simulink model "power_supply"  (R2023b)
settings: Solver=ode1  StartTime=0.0  StopTime=0.16  FixedStep=Ts  MaxStep=1e-6  RelTol=1e-4  EnableMultiTasking=on
values from neighbouring files (symbols this model uses):
  ca = 36e-6    (= 3.6e-05)    [parameters.m]
  cd = 2000e-6    (= 0.002)    [parameters.m]
  ckz = 1.2e-6    (= 1.2e-06)    [parameters.m]
  cs = 7720e-6    (= 0.00772)    [parameters.m]
  E = 512    [parameters.m]
  Kp1 = 0.2    [parameters.m]
  Kp2 = 2.22    [parameters.m]
  La = 0.1e-3    (= 0.0001)    [parameters.m]
  Ld = 0.3e-3    (= 0.0003)    [parameters.m]
  Lk = 2e-3    (= 0.002)    [parameters.m]
  Lm2 = 21e-3    (= 0.021)    [parameters.m]
  Ls = 0.7e-3    (= 0.0007)    [parameters.m]
  Ra = 0.01    [parameters.m]
  Rk = 19.2    [parameters.m]
  Rm2 = 20    [parameters.m]
  Rs = 0.12    [parameters.m]
  Vref = 1    [parameters.m]
  Wpi = 1    [parameters.m]
  Wsm = 1    [parameters.m]
libraries: spsSeriesRLCBranchLib x24, spsLinearTransformerLib x6, spsVoltageMeasurementLib x3, spsCurrentMeasurementLib x2, spsUniversalBridgeLib x2, spsControlledVoltageSourceLib x1, simulink x1, slpidlib x1, spsPWMGenerator2LevelLib x1, spsVariableResistorLib x1, spspowerguiLib x1
settings Model: Creator=Danil  LastModifiedBy=lyapunov
settings SolverCC: MaxConsecutiveMinStep=2  ZeroCrossControl=DisableAll  AlgebraicLoopSolver=TrustRegion  SolverResetMethod=Robust
settings DataIOCC: LimitDataPoints=on  SaveFormat=Array  ReturnWorkspaceOutputs=off
settings OptimizationCC: LifeSpan=inf
settings DebuggingCC: UnderspecifiedInitializationDetection=Classic  MergeDetectMultiDrivingBlocksExec=none  SolverPrmCheckMsg=warning  SFUnexpectedBacktrackingDiag=warning  SFNoUnconditionalDefaultTransitionDiag=warning  SFExecutionAtInitializationDiag=none  ArithmeticOperatorsInVariantConditions=warning
settings HardwareCC: ProdBitPerPointer=32  ProdBitPerSizeT=32  ProdBitPerPtrDiffT=32  ProdLargestAtomicFloat=None  ProdIntDivRoundTo=Undefined  ProdEndianess=Unspecified  ProdWordSize=32  ProdHWDeviceType=32-bit Generic
settings ModelReferenceCC: EnableRefExpFcnMdlSchedulingChecks=on  PropagateSignalLabelsOutOfModel=off
settings SFSimCC: SimUseLocalCustomCode=off  CustomCodeUndefinedFunction=UseInterfaceOnly
settings RTWCC: RTWUseLocalCustomCode=off  DLArmComputeVersion=19.05
settings CodeAppCC: StateflowObjectComments=on
settings GRTTargetCC: TargetLangStandard=C89/C90 (ANSI)
settings ConfigComp: CovMetricSettings=dw  CovSaveCumulativeToWorkspaceVar=on  CovSaveSingleToWorkspaceVar=on  CovExternalEMLEnable=off
settings SimscapeCC: SimscapeNormalizeSystem=off

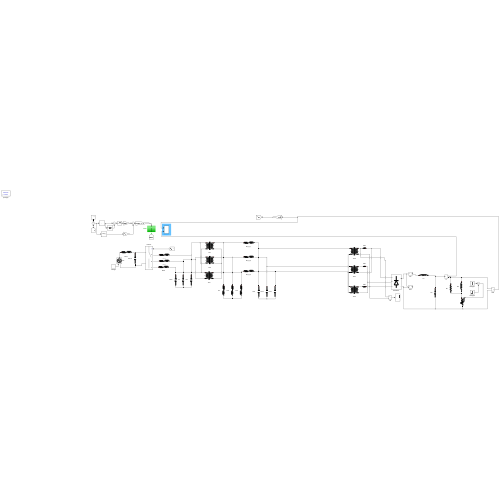
[thumbnail: Simulink's stored preview of the top-level diagram]
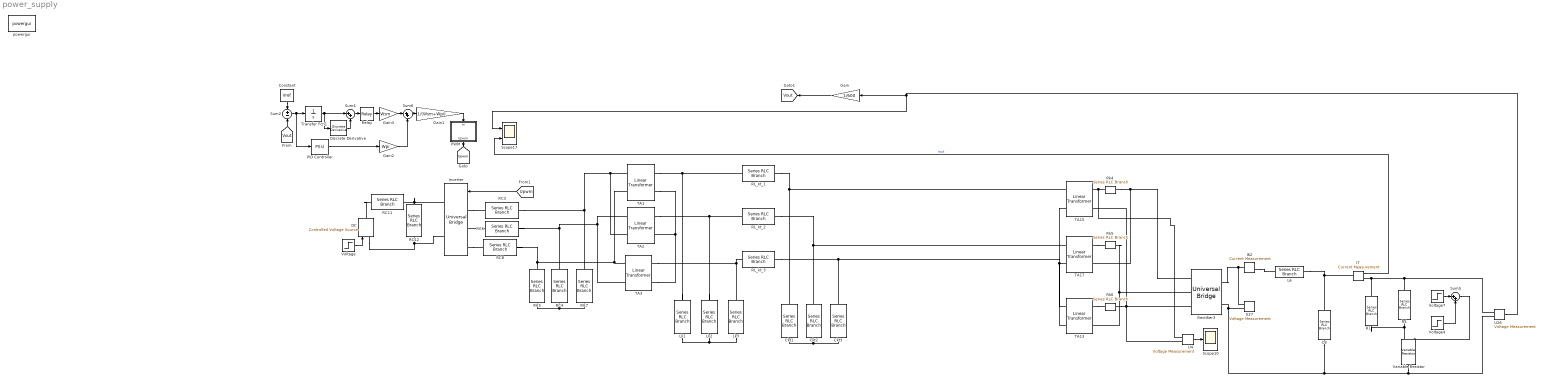
== system power_supply ==
  C8 : spsSeriesRLCBranchLib/Series RLC Branch  LConnTagsString=__new0  RConnTagsString=__new0  BranchType=C  Resistance=0.001  Inductance=1e-3  SetiL0=off  InitialCurrent=0  Capacitance=cd  Setx0=off  InitialVoltage=330  Measurements=None
  Ckt1 : spsSeriesRLCBranchLib/Series RLC Branch  LConnTagsString=__new0  RConnTagsString=__new0  BranchType=C  Resistance=1e-3  Inductance=1e-3  SetiL0=off  InitialCurrent=0  Capacitance=ckz  Setx0=off  InitialVoltage=0  Measurements=None
  Ckt2 : spsSeriesRLCBranchLib/Series RLC Branch  LConnTagsString=__new0  RConnTagsString=__new0  BranchType=C  Resistance=1e-3  Inductance=1e-3  SetiL0=off  InitialCurrent=0  Capacitance=ckz  Setx0=off  InitialVoltage=0  Measurements=None
  Ckt3 : spsSeriesRLCBranchLib/Series RLC Branch  LConnTagsString=__new0  RConnTagsString=__new0  BranchType=C  Resistance=1e-3  Inductance=1e-3  SetiL0=off  InitialCurrent=0  Capacitance=ckz  Setx0=off  InitialVoltage=0  Measurements=None
  Constant : Constant  Value=Vref
  DC : spsControlledVoltageSourceLib/Controlled Voltage Source  Initialize=on  Source_Type=AC  Amplitude=0  Phase=0  Frequency=0  Measurements=None
  Discrete Derivative : simulink/Discrete/Discrete Derivative  gainval=K  ICPrevScaledInput=0.0  OutMin=[]  OutMax=[]  OutDataType=fixdt(1, 16)  OutScaling=2^-10  DoSatur=off
  Gain : Gain  Gain=1/600
  Gain1 : Gain  Gain=1/(Wsm+Wpi)
  Gain2 : Gain  Gain=Wpi
  Gain3 : Gain  Gain=Wsm
  I62 : spsCurrentMeasurementLib/Current Measurement  PhasorSimulation=off  OutputType=Complex  PSBequivalent=0
  I7 : spsCurrentMeasurementLib/Current Measurement  PhasorSimulation=off  OutputType=Complex  PSBequivalent=0
  Inverter : spsUniversalBridgeLib/Universal Bridge  Arms=3  SnubberResistance=1e9  SnubberCapacitance=inf  Device=Ideal Switches  Ron=1e-4  Lon=0  ForwardVoltages="[  0  0  ]"  ForwardVoltage=0  GTOparameters=[ 10e-6 , 20e-6 ]  IGBTparameters=[ 1e-6 , 2e-6 ]  Measurements=None  Measurements_2=None  converterType=Rectifier
  L6 : spsSeriesRLCBranchLib/Series RLC Branch  LConnTagsString=__new0  RConnTagsString=__new0  BranchType=L  Resistance=1  Inductance=Ld  SetiL0=off  InitialCurrent=0  Capacitance=3*560e-6  Setx0=off  InitialVoltage=330  Measurements=Branch voltage
  Lk1 : spsSeriesRLCBranchLib/Series RLC Branch  LConnTagsString=__new0  RConnTagsString=__new0  BranchType=RL  Resistance=Rm2  Inductance=Lm2  SetiL0=off  InitialCurrent=0  Capacitance=2e-6  Setx0=off  InitialVoltage=0  Measurements=None
  Lk2 : spsSeriesRLCBranchLib/Series RLC Branch  LConnTagsString=__new0  RConnTagsString=__new0  BranchType=RL  Resistance=Rm2  Inductance=Lm2  SetiL0=off  InitialCurrent=0  Capacitance=2e-6  Setx0=off  InitialVoltage=0  Measurements=None
  Lk3 : spsSeriesRLCBranchLib/Series RLC Branch  LConnTagsString=__new0  RConnTagsString=__new0  BranchType=RL  Resistance=Rm2  Inductance=Lm2  SetiL0=off  InitialCurrent=0  Capacitance=2e-6  Setx0=off  InitialVoltage=0  Measurements=None
  PID Controller : slpidlib/PID Controller  Controller=PI  Form=Parallel  TimeDomain=Continuous-time  UseExternalTs=off  SampleTime=-1  IntegratorMethod=Forward Euler  FilterMethod=Forward Euler  ControllerParametersSource=internal  P=1.00507485861724  I=150.819020908144  UseKiTs=off  D=-0.000448447036645532  N=378.094165182863  UseFilter=on  TunerSelectOption=Transfer Function Based (PID Tuner App)  InitialConditionSource=internal  InitialConditionForIntegrator=0  InitialConditionForFilter=0  DifferentiatorICPrevScaledInput=0  ExternalReset=none  TrackingMode=off  Kt=1  LimitOutput=off  SatLimitsSource=internal  UpperSaturationLimit=inf  LowerSaturationLimit=-inf  LinearizeAsGain=on  AntiWindupMode=none  Kb=1  LimitIntegrator=off  UpperIntegratorSaturationLimit=inf  LowerIntegratorSaturationLimit=-inf  POutMin=[]  POutMax=[]  IOutMin=[]  IOutMax=[]  DOutMin=[]  DOutMax=[]  NOutMin=[]  NOutMax=[]  SumOutMin=[]  SumOutMax=[]  SaturationOutMin=[]  SaturationOutMax=[]  PParamMin=[]  PParamMax=[]  IParamMin=[]  IParamMax=[]  DParamMin=[]  DParamMax=[]  NParamMin=[]  NParamMax=[]  KbParamMin=[]  KbParamMax=[]  KtParamMin=[]  KtParamMax=[]  KbOutMin=[]  KbOutMax=[]  KtOutMin=[]  KtOutMax=[]  IntegratorOutMin=[]  IntegratorOutMax=[]  FilterOutMin=[]  FilterOutMax=[]  SumI1OutMin=[]  SumI1OutMax=[]  SumI2OutMin=[]  SumI2OutMax=[]  SumI3OutMin=[]  SumI3OutMax=[]  SumI4OutMin=[]  SumI4OutMax=[]  SumDOutMin=[]  SumDOutMax=[]  DifferentiatorOutMin=[]  DifferentiatorOutMax=[]  FilterDiffOutCoefMin=[]  FilterDiffOutCoefMax=[]  ReciprocalOutMin=[]  ReciprocalOutMax=[]  SumDenOutMin=[]  SumDenOutMax=[]  SumNumOutMin=[]  SumNumOutMax=[]  DivideOutMin=[]  DivideOutMax=[]  UdiffTsProdOutMin=[]  UdiffTsProdOutMax=[]  NTsProdOutMin=[]  NTsProdOutMax=[]  UintegralTsProdOutMin=[]  UintegralTsProdOutMax=[]  UngainTsProdOutMin=[]  UngainTsProdOutMax=[]  ClampingZeroOutDataTypeStr=Inherit: Inherit via back propagation  ClampingZeroOutMin=[]  ClampingZeroOutMax=[]  FilterDenConstantOutDataTypeStr=Inherit: Inherit via back propagation  FilterDenConstantOutMin=[]  FilterDenConstantOutMax=[]  PCopyOutDataTypeStr=Inherit: Inherit via back propagation  PCopyOutMin=[]  PCopyOutMax=[]  NCopyOutDataTypeStr=Inherit: Inherit via back propagation  NCopyOutMin=[]  NCopyOutMax=[]  IntegratorContinuousStateAttributes=''  IntegratorStateMustResolveToSignalObject=off  IntegratorRTWStateStorageClass=Auto  FilterContinuousStateAttributes=''  FilterStateMustResolveToSignalObject=off  FilterRTWStateStorageClass=Auto  ParallelPVariant=InternalParameters  IdealPVariant=Disabled  IVariant=InternalParameters  DVariant=Disabled  IntegratorVariant=Continuous  SatVariant=Disabled  AWVariant=Passthrough  PCopyVariant=Disabled  TRVariant=Disabled  FdbkBlocksVariant=Forward  IdealPFdbkVariant=Disabled  SatFdbkVariant=Disabled  DerivativeFilterVariant=Disabled  NVariant=Disabled  NCopyVariant=Disabled_SignalSpec  FilterICVariant=Disabled  IntegratorICVariant=InternalICs  ExternalResetVariant=Disabled  TRSumVariant=Passthrough  SumFdbkVariant=Disabled  SumVariant=Sum_PI  TsampFilterVariant=InternalTs  TsampNgainVariant=Passthrough  TsampIntegralVariant=Disabled_SignalSpec  ExternalSaturationOutDataTypeStr=Inherit: Same as second input
  PWM : Subsystem
  R1 : spsSeriesRLCBranchLib/Series RLC Branch  LConnTagsString=__new0  RConnTagsString=__new0  BranchType=R  Resistance=1e6  Inductance=0.67e-3  SetiL0=off  InitialCurrent=0  Capacitance=0.2775e-6  Setx0=off  InitialVoltage=0  Measurements=Branch voltage and current
  R4 : spsSeriesRLCBranchLib/Series RLC Branch  LConnTagsString=__new0  RConnTagsString=__new0  BranchType=L  Resistance=7.66+0.766  Inductance=0.67e-3  SetiL0=off  InitialCurrent=0  Capacitance=0.2775e-6  Setx0=off  InitialVoltage=0  Measurements=Branch voltage and current
  RC11 : spsSeriesRLCBranchLib/Series RLC Branch  LConnTagsString=__new0  RConnTagsString=__new0  BranchType=RL  Resistance=Rs  Inductance=Ls  SetiL0=off  InitialCurrent=0  Capacitance=6e-6  Setx0=off  InitialVoltage=0  Measurements=None
  RC12 : spsSeriesRLCBranchLib/Series RLC Branch  LConnTagsString=__new0  RConnTagsString=__new0  BranchType=C  Resistance=Rk  Inductance=Lk  SetiL0=off  InitialCurrent=0  Capacitance=cs  Setx0=off  InitialVoltage=0  Measurements=None
  RC3 : spsSeriesRLCBranchLib/Series RLC Branch  LConnTagsString=__new0  RConnTagsString=__new0  BranchType=RL  Resistance=Ra  Inductance=La  SetiL0=off  InitialCurrent=0  Capacitance=6e-6  Setx0=off  InitialVoltage=0  Measurements=None
  RC4 : spsSeriesRLCBranchLib/Series RLC Branch  LConnTagsString=__new0  RConnTagsString=__new0  BranchType=C  Resistance=Rk  Inductance=Lk  SetiL0=off  InitialCurrent=0  Capacitance=ca  Setx0=off  InitialVoltage=0  Measurements=None
  RC5 : spsSeriesRLCBranchLib/Series RLC Branch  LConnTagsString=__new0  RConnTagsString=__new0  BranchType=C  Resistance=Rk  Inductance=Lk  SetiL0=off  InitialCurrent=0  Capacitance=ca  Setx0=off  InitialVoltage=0  Measurements=None
  RC6 : spsSeriesRLCBranchLib/Series RLC Branch  LConnTagsString=__new0  RConnTagsString=__new0  BranchType=RL  Resistance=Ra  Inductance=La  SetiL0=off  InitialCurrent=0  Capacitance=6e-6  Setx0=off  InitialVoltage=0  Measurements=None
  RC7 : spsSeriesRLCBranchLib/Series RLC Branch  LConnTagsString=__new0  RConnTagsString=__new0  BranchType=C  Resistance=Rk  Inductance=Lk  SetiL0=off  InitialCurrent=0  Capacitance=ca  Setx0=off  InitialVoltage=0  Measurements=None
  RC8 : spsSeriesRLCBranchLib/Series RLC Branch  LConnTagsString=__new0  RConnTagsString=__new0  BranchType=RL  Resistance=Ra  Inductance=La  SetiL0=off  InitialCurrent=0  Capacitance=6e-6  Setx0=off  InitialVoltage=0  Measurements=None
  RL_kt_1 : spsSeriesRLCBranchLib/Series RLC Branch  LConnTagsString=__new0  RConnTagsString=__new0  BranchType=RL  Resistance=Rk  Inductance=Lk  SetiL0=off  InitialCurrent=0  Capacitance=1e-6  Setx0=off  InitialVoltage=0  Measurements=None
  RL_kt_2 : spsSeriesRLCBranchLib/Series RLC Branch  LConnTagsString=__new0  RConnTagsString=__new0  BranchType=RL  Resistance=Rk  Inductance=Lk  SetiL0=off  InitialCurrent=0  Capacitance=1e-6  Setx0=off  InitialVoltage=0  Measurements=None
  RL_kt_3 : spsSeriesRLCBranchLib/Series RLC Branch  LConnTagsString=__new0  RConnTagsString=__new0  BranchType=RL  Resistance=Rk  Inductance=Lk  SetiL0=off  InitialCurrent=0  Capacitance=1e-6  Setx0=off  InitialVoltage=0  Measurements=None
  Rectifier3 : spsUniversalBridgeLib/Universal Bridge  Arms=3  SnubberResistance=1e9  SnubberCapacitance=inf  Device=Diodes  Ron=1e-4  Lon=0  ForwardVoltages="[  0  0  ]"  ForwardVoltage=1.2  GTOparameters=[ 10e-6 , 20e-6 ]  IGBTparameters=[ 1e-6 , 2e-6 ]  Measurements=None  Measurements_2=None  converterType=Rectifier
  Relay : Relay  OnSwitchValue=0.01  OffSwitchValue=-0.01
  Rk4 : spsSeriesRLCBranchLib/Series RLC Branch  LConnTagsString=__new0  RConnTagsString=__new0  BranchType=R  Resistance=1e-7  Inductance=10e-3  SetiL0=off  InitialCurrent=0  Capacitance=3*560e-6  Setx0=off  InitialVoltage=330  Measurements=None
  Rk5 : spsSeriesRLCBranchLib/Series RLC Branch  LConnTagsString=__new0  RConnTagsString=__new0  BranchType=R  Resistance=1e-7  Inductance=10e-3  SetiL0=off  InitialCurrent=0  Capacitance=3*560e-6  Setx0=off  InitialVoltage=330  Measurements=None
  Rk6 : spsSeriesRLCBranchLib/Series RLC Branch  LConnTagsString=__new0  RConnTagsString=__new0  BranchType=R  Resistance=1e-7  Inductance=10e-3  SetiL0=off  InitialCurrent=0  Capacitance=3*560e-6  Setx0=off  InitialVoltage=330  Measurements=None
  Scope10 : Scope
  Scope17 : Scope  NumInputPorts=2
  Sum2 : Sum  Inputs=+-
  Sum4 : Sum  Inputs=|++
  Sum5 : Sum  Inputs=|++
  Sum6 : Sum  Inputs=|++
  TA1 : spsLinearTransformerLib/Linear Transformer  UNITS=SI  NominalPower=[50e3 1000 ]  winding1=[1 0 0]  winding2=[1/Kp1 0 0]  ThreeWindings=off  winding3=[3.15e+05 9922.5 63.169]  RmLm=[1e6 1e6]  Measurements=None  DataType=on
  TA13 : spsLinearTransformerLib/Linear Transformer  UNITS=SI  NominalPower=[50e3 1000 ]  winding1=[220 0 0]  winding2=[220/Kp2 0 0]  ThreeWindings=off  winding3=[3.15e+05 9922.5 63.169]  RmLm=[1e6 1e6]  Measurements=None  DataType=on
  TA15 : spsLinearTransformerLib/Linear Transformer  UNITS=SI  NominalPower=[50e3 1000 ]  winding1=[220 0 0]  winding2=[220/Kp2 0 0]  ThreeWindings=off  winding3=[3.15e+05 9922.5 63.169]  RmLm=[1e6 1e6]  Measurements=None  DataType=on
  TA17 : spsLinearTransformerLib/Linear Transformer  UNITS=SI  NominalPower=[50e3 1000 ]  winding1=[220 0 0]  winding2=[220/Kp2 0 0]  ThreeWindings=off  winding3=[3.15e+05 9922.5 63.169]  RmLm=[1e6 1e6]  Measurements=None  DataType=on
  TA2 : spsLinearTransformerLib/Linear Transformer  UNITS=SI  NominalPower=[50e3 1000 ]  winding1=[1 0 0]  winding2=[1/Kp1 0 0]  ThreeWindings=off  winding3=[3.15e+05 9922.5 63.169]  RmLm=[1e6 1e6]  Measurements=None  DataType=on
  TA3 : spsLinearTransformerLib/Linear Transformer  UNITS=SI  NominalPower=[50e3 1000 ]  winding1=[1 0 0]  winding2=[1/Kp1 0 0]  ThreeWindings=off  winding3=[3.15e+05 9922.5 63.169]  RmLm=[1e6 1e6]  Measurements=None  DataType=on
  Transfer Fcn1 : TransferFcn  Denominator=[1 0]
  U26 : spsVoltageMeasurementLib/Voltage Measurement  PhasorSimulation=off  OutputType=Complex  PSBequivalent=0
  U27 : spsVoltageMeasurementLib/Voltage Measurement  PhasorSimulation=off  OutputType=Complex  PSBequivalent=0
  U4 : spsVoltageMeasurementLib/Voltage Measurement  PhasorSimulation=off  OutputType=Complex  PSBequivalent=0
  Variable Resistor : spsVariableResistorLib/Variable Resistor  Rabsmin=1e-3
      settings: LibrarySourceBlock=sps_lib/Passives/Variable Resistor
  Voltage : Step  Time=0  After=E  SampleTime=0
  Voltage4 : Step  Time=0.12  After=0.2*7.66  SampleTime=0
  Voltage7 : Step  Time=0.07  Before=7.66  After=0.9*7.66  SampleTime=0
  powergui : spspowerguiLib/powergui  Priority=1  SimulationMode=Discrete  SampleTime=1e-6  frequency=60  Iterations=50  frequencyindice=0  Pbase=100e6  ErrMax=1e-4  UnitsV=kV  UnitsW=MW  buscounter=0  FunctionMessages=on  echomessages=off  EnableUseOfTLC=off  CurrentSourceSwitches=off  DisableSnubberDevices=off  DisableRonSwitches=off  DisableVfSwitches=off  DisplayEquations=off  AutomaticDiscreteSolvers=off  SolverType=Backward Euler  Interpol=off  ExternalGateDelay=off  methode=off  Ts=0  x0status=zero  SPID=off  SwTol=0  HookPort=off  NonlinearTolerance=1e-4  nMaxIteration=100  ContinueOnMaxIteration=off  RestoreLinks=warning  ResistiveCurrentMeasurement=off  Frange=[0:2:500]  Ylog=off  Xlog=on  ShowGrid=off  save=off  variable=ZData  structure=Uvyh  ZoomFFT=on  StartTime=0.02  cycles=5  DisplayStyle=2  fundamental=1000  FreqAxis=off  MaxFrequency=100000  frequencyindicesteady=1000  RmsSteady=1  display=off
  tag scope: Upwm=global, Vout=global
  wires:
  PWM/1(Upwm) -> [Upwm]
  Voltage/1 -> DC/1
  U4/1 -> Scope10/1
  Voltage7/1 -> Sum5/1
  Sum5/1 -> Variable Resistor/1
  Voltage4/1 -> Sum5/2
  U26/1 -> Scope17/1, Gain/1
  I7/1 -> Scope17/2  "Iout"
  Transfer Fcn1/1 -> Sum4/1, Discrete Derivative/1
  Discrete Derivative/1 -> Sum4/2
  Sum4/1 -> Relay/1
  Sum2/1 -> PID Controller/1, Transfer Fcn1/1
  Relay/1 -> Gain3/1
  Sum6/1 -> Gain1/1
  Gain2/1 -> Sum6/2
  Gain3/1 -> Sum6/1
  PID Controller/1 -> Gain2/1
  Gain1/1 -> PWM/1(In)
  Constant/1 -> Sum2/1
  Gain/1 -> [Vout]
  [Vout] -> Sum2/2
  [Upwm] -> Inverter/1
  connections:
  Rectifier3/RConn1 -- I62/LConn1 -- U27/LConn1
  RL_kt_3/RConn1 -- TA13/LConn1 -- Ckt3/LConn1
  TA17/RConn1 -- Rk5/RConn1
  TA15/RConn2 -- U4/LConn2 -- Rectifier3/LConn3 -- Rk6/LConn1
  Lk1/LConn1 -- RL_kt_1/LConn1 -- TA1/RConn1
  TA17/RConn2 -- Rectifier3/LConn1 -- Rk4/LConn1
  Lk2/LConn1 -- TA2/RConn1 -- RL_kt_2/LConn1
  Lk3/LConn1 -- TA3/RConn1 -- RL_kt_3/LConn1
  RC12/RConn1 -- DC/LConn1 -- Inverter/RConn2
  RC12/LConn1 -- Inverter/RConn1 -- RC11/RConn1
  U26/LConn2 -- Variable Resistor/RConn1 -- C8/RConn1 -- U27/LConn2 -- Rectifier3/RConn2
  RL_kt_2/RConn1 -- TA17/LConn1 -- Ckt2/LConn1
  Lk1/RConn1 -- Lk3/RConn1 -- Lk2/RConn1
  Ckt3/RConn1 -- Ckt1/RConn1 -- Ckt2/RConn1
  TA15/RConn1 -- U4/LConn1 -- Rk4/RConn1
  Rk5/LConn1 -- Rectifier3/LConn2 -- TA13/RConn2
  TA13/RConn1 -- Rk6/RConn1
  I62/RConn1 -- L6/LConn1
  TA1/RConn2 -- TA3/RConn2 -- TA2/RConn2
  RC7/RConn1 -- RC5/RConn1 -- RC4/RConn1
  C8/LConn1 -- I7/LConn1 -- L6/RConn1
  RC11/LConn1 -- DC/RConn1
  RL_kt_1/RConn1 -- TA15/LConn1 -- Ckt1/LConn1
  U26/LConn1 -- R4/LConn1 -- R1/LConn1 -- I7/RConn1
  TA3/LConn1 -- RC8/RConn1 -- RC5/LConn1 -- TA1/LConn2
  TA15/LConn2 -- TA13/LConn2 -- TA17/LConn2
  TA2/LConn2 -- RC3/RConn1 -- RC7/LConn1 -- TA1/LConn1
  TA3/LConn2 -- TA2/LConn1 -- RC6/RConn1 -- RC4/LConn1
  Inverter/LConn1 -- RC3/LConn1
  RC6/LConn1 -- Inverter/LConn2
  Inverter/LConn3 -- RC8/LConn1
  Variable Resistor/LConn1 -- R1/RConn1 -- R4/RConn1

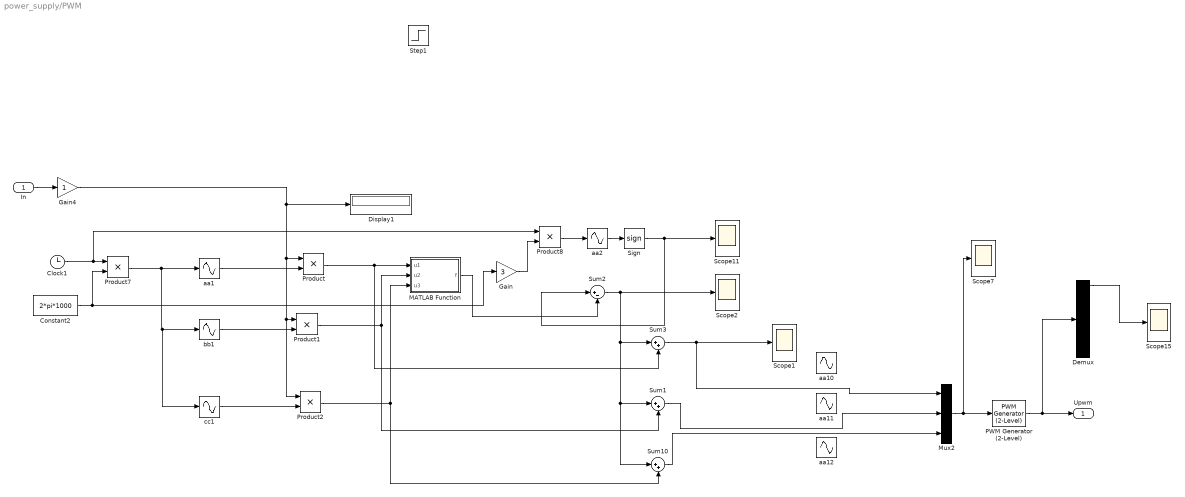
== system power_supply/PWM ==
  In : Inport
  Clock1 : Clock
  Constant2 : Constant  Value=2*pi*1000
  Demux : Demux  Outputs=6
  Display1 : Display
  Gain : Gain  Gain=3
  Gain4 : Gain
  MATLAB Function : MATLAB Function  TreatAsAtomicUnit=on
  Mux2 : Mux  Inputs=3
  PWM Generator (2-Level) : spsPWMGenerator2LevelLib/PWM Generator (2-Level)  ModulatorType=Three-phase bridge (6 pulses)  ModulatorMode=Unsynchronized  Fc=48000  Pc=90  nF=27  MinMax="[ -1  1 ]"  SamplingTechnique=Natural  ModulatingSignals=off  m=0.8  Freq=60  Phase=0  Ts=1e-6  ShowCarrierOutport=off
  Product{,1..2,7..8} (5 alike) : Product
  Scope{1..2,7,11,15} (5 alike) : Scope
  Sign : Signum
  Step1 : Step  Time=0.16  After=-0.03  SampleTime=0
  Sum1 : Sum  Inputs=|++
  Sum10 : Sum  Inputs=|++
  Sum2 : Sum  Inputs=|+-
  Sum3 : Sum  Inputs=|++
  aa1 : Sin  TimeSource=Use external signal  Amplitude=1/cos(pi/6)  SampleTime=0
  aa10 : Sin  Frequency=2*pi*1000  SampleTime=0
  aa11 : Sin  Frequency=2*pi*1000  Phase=-2*pi/3  SampleTime=0
  aa12 : Sin  Frequency=2*pi*1000  Phase=2*pi/3  SampleTime=0
  aa2 : Sin  TimeSource=Use external signal  Phase=-pi  SampleTime=0
  bb1 : Sin  TimeSource=Use external signal  Amplitude=1/cos(pi/6)  Phase=-2*pi/3  SampleTime=0
  cc1 : Sin  TimeSource=Use external signal  Amplitude=1/cos(pi/6)  Phase=2*pi/3  SampleTime=0
  Upwm : Outport
  wires:
  Mux2/1 -> PWM Generator (2-Level)/1, Scope7/1
  Demux/1 -> Scope15/1
  Product1/1 -> MATLAB Function/2(u2), Sum1/2
  Product2/1 -> MATLAB Function/3(u3), Sum10/2
  MATLAB Function/1(f) -> Sum2/2
  Product/1 -> Sum3/2, MATLAB Function/1(u1)
  Sign/1 -> Sum2/1, Scope11/1
  Sum2/1 -> Sum10/1, Sum1/1, Sum3/1, Scope2/1
  aa1/1 -> Product/2
  bb1/1 -> Product1/2
  cc1/1 -> Product2/2
  aa2/1 -> Sign/1
  Constant2/1 -> Product7/2, Gain/1
  Product7/1 -> cc1/1, bb1/1, aa1/1
  Clock1/1 -> Product8/1, Product7/1
  Product8/1 -> aa2/1
  Gain/1 -> Product8/2
  Sum3/1 -> Mux2/1, Scope1/1
  Sum1/1 -> Mux2/2
  Sum10/1 -> Mux2/3
  PWM Generator (2-Level)/1 -> Upwm/1, Demux/1
  In/1 -> Gain4/1
  Gain4/1 -> Display1/1, Product2/1, Product1/1, Product/1

== matlab function power_supply/PWM/MATLAB Function ==
  data: u1 input; f output; u2 input; u3 input
function f = myfun(u1,u2,u3)
if (abs(u1) > abs(u2))&&(abs(u1) > abs(u3))
    f= u1;
elseif (abs(u2) > abs(u3))&& (abs(u2)> abs(u1))  
    f = u2;
    else 
        f = u3;
    end
